simulink model "pddob"  (Simulink 4.00)
settings: Solver=ode45  StartTime=0.0  StopTime=100.0  RelTol=1e-3
values from neighbouring files (symbols this model uses):
  B = 1.8062    [para_pdwithfriction.m]
  J = 1.386    [para_pdwithfriction.m]
  Kp = 4    [para_pdwithfriction.m]
  Kv = 0.02    [para_pdwithfriction.m]
  lqden = [1,-1.99952441809169,0.99952465041253,0,0,0]    [para_pdwithfriction.m]
  lqnum = [1295.1607010647958,-3697.4382459623394,2121.2993486042033,2870.2528627401011,-3790.4537725173027,1201.1791063028616]    [para_pdwithfriction.m]
  ts = 0.001    [para_pdwithfriction.m]
undefined symbols (not defined in the file or in its folder): F_step, g2den, g2num, qzden, qznum
libraries: simulink3 x1
settings Model: LastModifiedBy=liuyuan1  MaxDataPoints=100000  ExtModeTrigMode=oneshot  ExtModeArmWhenConnect=off

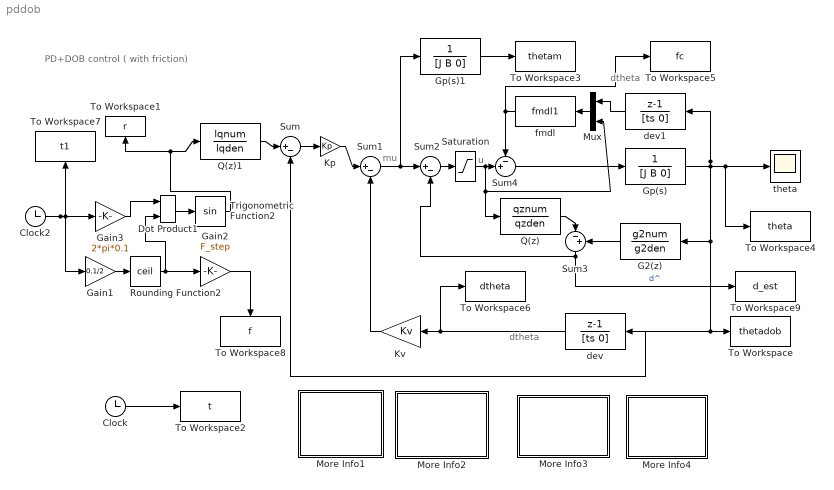
== system pddob ==
  note: dtheta
  note: u
  note: PD+DOB control ( with friction)
  note: dtheta
  note: mu
  " Kv" : Gain  Orientation=left  Gain=Kv  Multiplication=Element-wise(K.*u)  SaturateOnIntegerOverflow=on
  Clock : Clock
      settings: DisplayTime=off  Decimation=10
  Clock2 : Clock
      settings: Decimation=10
  Dot Product1 : simulink3/Math/Dot Product
  G2(z) : DiscreteTransferFcn  Orientation=left  Numerator=g2num  Denominator=g2den  SampleTime=0.001  Realization=auto
      settings: RTWStateStorageClass=Auto
  Gain1 : Gain  Gain=0.1/2  Multiplication=Element-wise(K.*u)  SaturateOnIntegerOverflow=on
  Gain2 : Gain  Gain=F_step  Multiplication=Element-wise(K.*u)  SaturateOnIntegerOverflow=on
  Gain3 : Gain  Gain=2*pi*0.1  Multiplication=Element-wise(K.*u)  SaturateOnIntegerOverflow=on
  Gp(s) : TransferFcn  Numerator=[0 0 1]  Denominator=[J B 0]  AbsoluteTolerance=auto  Realization=auto
  Gp(s)1 : TransferFcn  Numerator=[0 0 1]  Denominator=[J B 0]  AbsoluteTolerance=auto  Realization=auto
  "Kp " : Gain  Gain=Kp  Multiplication=Element-wise(K.*u)  SaturateOnIntegerOverflow=on
  More Info1 : Subsystem
      settings: OpenFcn=eval(['paradob']);  RTWFcnNameOpts=Auto  RTWFileNameOpts=Auto
      mask Display: disp('Double click\nhere for\nload parameters')
  More Info2 : Subsystem
      settings: OpenFcn=eval(['postpdwithfriction']);  RTWFcnNameOpts=Auto  RTWFileNameOpts=Auto
      mask Display: disp('Double click\nhere for plot')
  More Info3 : Subsystem
      settings: OpenFcn=eval(['test_freq']);  RTWFcnNameOpts=Auto  RTWFileNameOpts=Auto
      mask Display: disp('Double click\nhere for \ncompute frequency')
  More Info4 : Subsystem
      settings: OpenFcn=eval(['bode_plot']);  RTWFcnNameOpts=Auto  RTWFileNameOpts=Auto
      mask Display: disp('Double click\nhere for \ndraw bode')
  Mux : Mux  Orientation=left  Inputs=2
  Q(z) : DiscreteTransferFcn  Numerator=qznum  Denominator=qzden  SampleTime=0.001  Realization=auto
      settings: RTWStateStorageClass=Auto
  Q(z)1 : DiscreteTransferFcn  Numerator=lqnum  Denominator=lqden  SampleTime=0.001  Realization=auto
      settings: RTWStateStorageClass=Auto
  Rounding Function2 : Rounding  Operator=ceil
  Saturation : Saturate  UpperLimit=10  LowerLimit=-10  LinearizeAsGain=on
  Sum : Sum  Inputs=|+-  SaturateOnIntegerOverflow=on
  Sum1 : Sum  Inputs=|+-  SaturateOnIntegerOverflow=on
  Sum2 : Sum  Inputs=|+-  SaturateOnIntegerOverflow=on
  Sum3 : Sum  Orientation=down  Inputs=|-+  SaturateOnIntegerOverflow=on
  Sum4 : Sum  Inputs=-+|  SaturateOnIntegerOverflow=on
  To Workspace : ToWorkspace  VariableName=thetadob  SampleTime=-1  SaveFormat=Array
      settings: MaxDataPoints=100000
  To Workspace1 : ToWorkspace  VariableName=r  SampleTime=-1  SaveFormat=Array
      settings: Orientation=up  MaxDataPoints=100000
  To Workspace2 : ToWorkspace  VariableName=t  SampleTime=-1  SaveFormat=Array
      settings: MaxDataPoints=100000
  To Workspace3 : ToWorkspace  VariableName=thetam  SampleTime=-1  SaveFormat=Array
      settings: MaxDataPoints=100000
  To Workspace4 : ToWorkspace  VariableName=theta  SampleTime=-1  SaveFormat=Array
      settings: MaxDataPoints=100000
  To Workspace5 : ToWorkspace  VariableName=fc  SampleTime=-1  SaveFormat=Array
      settings: MaxDataPoints=100000
  To Workspace6 : ToWorkspace  VariableName=dtheta  SampleTime=-1  SaveFormat=Array
      settings: MaxDataPoints=100000
  To Workspace7 : ToWorkspace  VariableName=t1  SampleTime=-1  SaveFormat=Array
      settings: Orientation=up
  To Workspace8 : ToWorkspace  VariableName=f  SampleTime=-1  SaveFormat=Array
      settings: Orientation=down  MaxDataPoints=100000
  To Workspace9 : ToWorkspace  VariableName=d_est  SampleTime=-1  SaveFormat=Array
      settings: MaxDataPoints=100000
  Trigonometric Function2 : Trigonometry  Operator=sin  OutputSignalType=auto
  dev : DiscreteTransferFcn  Orientation=left  Numerator=[1 -1]  Denominator=[ts 0]  SampleTime=0.001  Realization=auto
      settings: RTWStateStorageClass=Auto
  dev1 : DiscreteTransferFcn  Orientation=left  Numerator=[1 -1]  Denominator=[ts 0]  SampleTime=0.001  Realization=auto
      settings: RTWStateStorageClass=Auto
  fmdl : MATLABFcn  Orientation=left  MATLABFcn=fmdl1  OutputDimensions=-1  OutputSignalType=auto  Output1D=on
      settings: AttributesFormatString=fmdl2
  theta : Scope
      settings: TimeRange=auto  YMin=-1  YMax=1  SaveToWorkspace=off  SaveName=ScopeData  LimitDataPoints=on  MaxDataPoints=5000
  wires:
  Gp(s)/1 -> G2(z)/1, dev/1, Sum/2, To Workspace/1, dev1/1, theta/1, To Workspace4/1
  G2(z)/1 -> Sum3/2
  Q(z)/1 -> Sum3/1
  Sum/1 -> "Kp "/1
  "Kp "/1 -> Sum1/1
  " Kv"/1 -> Sum1/2
  Sum2/1 -> Saturation/1
  Sum4/1 -> Gp(s)/1
  Clock/1 -> To Workspace2/1
  Gp(s)1/1 -> To Workspace3/1
  Sum1/1 -> Sum2/1, Gp(s)1/1
  Sum3/1 -> To Workspace9/1, Sum2/2  "d^"
  fmdl/1 -> Sum4/1, To Workspace5/1
  Mux/1 -> fmdl/1
  dev1/1 -> Mux/1
  dev/1 -> " Kv"/1, To Workspace6/1
  Trigonometric Function2/1 -> To Workspace1/1, Q(z)1/1
  Clock2/1 -> Gain3/1, Gain1/1, To Workspace7/1
  Gain1/1 -> Rounding Function2/1
  Gain3/1 -> Dot Product1/1
  Dot Product1/1 -> Trigonometric Function2/1
  Rounding Function2/1 -> Dot Product1/2, Gain2/1
  Gain2/1 -> To Workspace8/1
  Q(z)1/1 -> Sum/1
  Saturation/1 -> Sum4/2, Q(z)/1, Mux/2

== system pddob/More Info1 ==

== system pddob/More Info2 ==

== system pddob/More Info3 ==

== system pddob/More Info4 ==
